simulink model "untitled"  (R2020a)
settings: Solver=VariableStepAuto  StartTime=0.0  StopTime=10.0  RelTol=1e-3
settings Model: Creator=dell  LastModifiedBy=dell

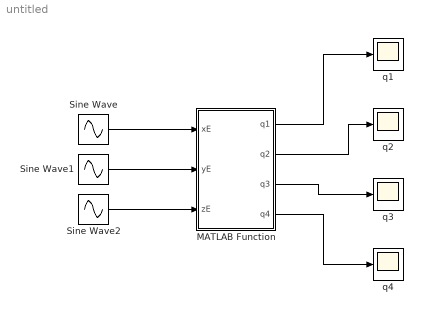
== system untitled ==
  MATLAB Function : MATLAB Function  TreatAsAtomicUnit=on
  Sine Wave : Sin  SampleTime=0
  Sine Wave1 : Sin  SampleTime=0
  Sine Wave2 : Sin  SampleTime=0
  q{1..4} (4 alike) : Scope
  wires:
  MATLAB Function/1(q1) -> q1/1
  MATLAB Function/2(q2) -> q2/1
  MATLAB Function/3(q3) -> q3/1
  MATLAB Function/4(q4) -> q4/1
  Sine Wave/1 -> MATLAB Function/1(xE)
  Sine Wave2/1 -> MATLAB Function/3(zE)
  Sine Wave1/1 -> MATLAB Function/2(yE)

== matlab function untitled/MATLAB Function ==
  data: xE input; q1 output; yE input; zE input; q2 output; q3 output; q4 output
function [q1,q2,q3,q4] = fcn(xE,yE,zE)
